simulink model "Udan_SOC"  (R2017b)
settings: Solver=FixedStepAuto  StartTime=0.0  StopTime=1000  FixedStep=0.1  RelTol=1e-3
values from neighbouring files (symbols this model uses):
  DenominatorOfIntegratorFactor = 100.0    [SOC_Stateflow.sldd]
  SOC_CalcSohLKT = 1.0    [SOC_Stateflow.sldd]
  SOC_CalcSOHTempLimit = 70.0    [SOC_Stateflow.sldd]
  SOC_CapPerCycle = 100.0    [SOC_Stateflow.sldd]
  SOC_CapTemp_HLimit = 200.0    [SOC_Stateflow.sldd]
  SOC_CapTemp_LLimit = 0.0    [SOC_Stateflow.sldd]
  Soc_ConfigInfo = 0    [SOC_Stateflow.sldd]
  SOC_DchgEndCalib = 0.0    [SOC_Stateflow.sldd]
  SOC_DiffVoltMin = 10.0    [SOC_Stateflow.sldd]
  SOC_DSOCJumpMax = 500.0    [SOC_Stateflow.sldd]
  SOC_EfficientHighLimit = 250.0    [SOC_Stateflow.sldd]
  SOC_EfficientLowLimit = 40.0    [SOC_Stateflow.sldd]
  SOC_EmptyAus = 0.0    [SOC_Stateflow.sldd]
  SOC_EnableOcv = 1.0    [SOC_Stateflow.sldd]
  SOC_END_CALIB_STATE : value not decoded    [SOC_Stateflow.sldd]
  SOC_HighRealSoc = 95.0    [SOC_Stateflow.sldd]
  SOC_LKTSohCycles = 0.0 1.0 10.0 20.0 30.0 40.0 50.0 60.0 70.0 80.0 90.0 100.0 110.0 120.0 130.0 140.0 150.0 160.0 170.0 180.0 190.0 200.0 210.0 220.0 230.0 240.0 250.0 260.0 270.0 280.0 290.0 300.0 310.0 320.0 330.0 340.0 350.0 360.0 370.0 380.0 390.0 400.0 410.0 420.0 430.0 440.0 450.0 460.0 470.0 480.0 490.0 500.0 510.0 520.0 530.0 540.0 550.0 560.0 570.0 580.0 590.0 600.0 610.0 620.0 630.0 640.0 650.0 660.0 670.0    [SOC_Stateflow.sldd]
  SOC_LKTSohTable = 1000.0 991.0 989.0 992.0 993.0 995.0 994.0 993.0 1000.0 997.0 1002.0 1000.0 992.0 1000.0 989.0 992.0 989.0 994.0 989.0 993.0 994.0 994.0 994.0 993.0 991.0 991.0 992.0 993.0 991.0 985.0 985.0 985.0 979.0 975.0 978.0 984.0 982.0 974.0 975.0 972.0 972.0 975.0 977.0 977.0 974.0 971.0 973.0 971.0 966.0 968.0 965.0 959.0 957.0 956.0 957.0 954.0 955.0 951.0 954.0 951.0 942.0 942.0 940.0 942.0 947.0 949.0    [SOC_Stateflow.sldd]
  SOC_LowRealSoc = 5.0    [SOC_Stateflow.sldd]
  SOC_NominalCap_AmS = 576000000.0    [SOC_Stateflow.sldd]
  SOC_NominalVol = 4000.0    [SOC_Stateflow.sldd]
  SOC_OCVTemp_HLimit = 106.0    [SOC_Stateflow.sldd]
  SOC_OCVTemp_LLimit = 29.0    [SOC_Stateflow.sldd]
  SOC_ShortCalibDSoc = 1.0    [SOC_Stateflow.sldd]
  SOC_SOCResolution = 10000.0    [SOC_Stateflow.sldd]
  SOC_SohCalcCapPercent = 8.0    [SOC_Stateflow.sldd]
  SOC_SohCalcHighLimit = 60.0    [SOC_Stateflow.sldd]
  SOC_SohCalcLowLimit = 10.0    [SOC_Stateflow.sldd]
  SOC_SohCalcMidLimit = 30.0    [SOC_Stateflow.sldd]
  SOC_SOHResolution = 1000.0    [SOC_Stateflow.sldd]
  SOC_State = <binary blob, 1163 chars, not shown>    [SOC_Stateflow.sldd]
  SOC_TempCap_CapBuffer : value not decoded    [SOC_Stateflow.sldd]
  SOC_TempCap_TempBuffer : value not decoded    [SOC_Stateflow.sldd]
  SocOcvCalib_ConfigInfo = 0.0    [SOC_Stateflow.sldd]
  SocOcvCalib_SocBuffer1 : value not decoded    [SOC_Stateflow.sldd]
  SocOcvCalib_TempBuffer : value not decoded    [SOC_Stateflow.sldd]
  SocOcvCalib_VoltageBuffer1 = 3300.0 3303.0 3305.0 3307.0 3310.0 3311.0 3313.0 3314.0 3316.0 3317.0 3319.0 3320.0 3322.0 3323.0 3325.0 3322.0 3323.0 3325.0 3310.0 3313.0 3315.0 3317.0 3320.0 3321.0 3323.0 3324.0 3326.0 3327.0 3329.0 3330.0 3332.0 3333.0 3335.0 3332.0 3333.0 3335.0 3320.0 3323.0 3325.0 3327.0 3330.0 3331.0 3333.0 3334.0 3336.0 3337.0 3339.0 3340.0 3342.0 3343.0 3345.0 3342.0 3343.0 3345.0 3330.0 3333.0 3335.0 3    [SOC_Stateflow.sldd]
  SOHCalibCycle = 10.0    [SOC_Stateflow.sldd]
undefined symbols (not defined in the file or in its folder): DatetimeM_GetReturnType, ParameterM_EeepParaIndexType, Soc_CumuLativeTypeType, SOC_EgthTempChgValue, Soc_EnergyBuffer, SOC_FithTempChgValue, SOC_FstSlowTempChgValue, SOC_FstTempChgValue, SOC_FthTempChgValue, SOC_MaxCap_AmS, SOC_SethTempChgValue, SOC_SixTempChgValue, SOC_SndSlowTempChgValue, SOC_SndTempChgValue, SOC_TrdSlowTempChgValue, SOC_TrdTempChgValue, SocDiagCalib_NoCalibReasonType
libraries: simulink x138, hdlsllib x24, dspindex x4
(part 9 of 10)

== matlab function Udan_SOC/SOC_Calculate/UdanSOCCalcn/LKTSOC/MATLAB Function2 ==
  data: cellTable input; enableOcv output; uCell input; diffVMin input; socBuffer input
function enableOcv = fcn(cellTable, uCell,diffVMin, socBuffer)
flag = uint8(0);
enableOcv = uint8(0);
for i = 1 : length(cellTable)-1
    if i == length(cellTable)
       flag = uint8(1);
    elseif uCell < cellTable(1)
           flag = uint8(1);
           break;
    else
           if cellTable(i)<=uCell && uCell < cellTable(i+1)
                break;
          end
    end
end
if flag < 1
    if i == 1 
        if cellTable(i+2) > cellTable(i+1) + uint16(diffVMin) && cellTable(i+1) > cellTable(i)+uint16(diffVMin) %% 压差大于10mv才认为区间有效
            flag = uint8(1);
        end
    elseif uCell >=cellTable(length(cellTable)) || socBuffer(i)>=10000
         flag = uint8(1);
    else
            if socBuffer(i+2)<=10000
                if cellTable(i+2) > cellTable(i+1) + uint16(diffVMin) && cellTable(i+1) > cellTable(i)+uint16(diffVMin) && cellTable(i) > cellTable(i-1)+uint16(diffVMin)
                    flag = uint8(1);
                end
            elseif socBuffer(i+1)<=10000
                if cellTable(i+1) > cellTable(i)+uint16(diffVMin) && cellTable(i) > cellTable(i-1)+uint16(diffVMin)
                    flag = uint8(1);
                end
            elseif socBuffer(i)<=10000
                if cellTable(i) > cellTable(i-1)+uint16(diffVMin)
                    flag = uint8(1);
                end
            else
                flag = uint8(1);
            end
    end
end

enableOcv = flag;

== matlab function Udan_SOC/SOC_Calculate/UdanSOCCalcn/Function-Call Subsystem4/Subsystem2/MATLAB Function2 ==
  data: input input; y output; bp input; table input
function y = interp_linear(input,bp,table)
data_type = class(table);
switch data_type
    case 'uint8'
        y = uint8(0);
    case 'uint16'
        y = uint16(0);
    case 'uint32'
        y = uint32(0);
end
if bp(1) == bp(2)
    y = table(2);
elseif length(bp) == length(table)
    if input <= bp(1)
        y = table(1);
    elseif input >= bp(end)
        y = table(end);
    else
        for i = 1 : length(bp)-1
            if input == bp(i)
                y = table(i);
                break;
            elseif input > bp(i) && input < bp(i+1)
                y = uint16(uint32(table(i)) - (uint32(table(i) - table(i+1)))*uint32((input-bp(i)))/uint32((bp(i+1)-bp(i))));
                break;
            else
            end
        end
    end
else
    msg = 'size dismatch';
    error(masg);
    y = 0;
end

== matlab function Udan_SOC/SOC_Calculate/UdanSOCCalcn/Function-Call Subsystem4/Subsystem2/MATLAB Function3 ==
  data: soh input; Cycles input; bp output; Table input; table output
function [bp,table] = fcn(soh, Cycles,Table)
    data_type = class(Table);
    uint8 index;
    index = GetSohLocationIndex(soh,Table);
    switch data_type
        case 'uint8'
            bp = uint8([Table(index+1) Table(index)]);
            table = GetDataType([Cycles(index) Cycles(index+1)]);
        case 'uint16'
            bp = uint16([Table(index+1) Table(index)]);
            table = GetDataType([Cycles(index) Cycles(index+1)]);
        case 'uint32'
            bp = uint32([Table(index+1) Table(index)]);
            table = GetDataType([Cycles(index) Cycles(index+1)]);
        otherwise
            bp = [ 0 0];
            table = [0 0];

    end
end
function ret = GetDataType(input)
    data_type1 = class(input);
    switch data_type1
        case 'uint8'
            ret = uint8([max(input) min(input)]);
        case 'uint16'
            ret = uint16([max(input) min(input)]);
        case 'uint32'
            ret = uint32([max(input) min(input)]);
        otherwise
            ret = [0 0];

    end
end

function index = GetSohLocationIndex(soh,sohTable)
    len = uint8(length(sohTable));
    i = uint8(0);
    index = uint8(1);
    if soh >= sohTable(1)
        index = uint8(1);
    elseif soh <= sohTable(len)
        index = len - 1;
    else
        for i = 1 : len - 1
            if soh <= sohTable(i) && soh>= sohTable(i+1)
                index = i;
                break;
            end
        end
    end
end

== stateflow chart Udan_SOC/SOC_Calculate/UdanSOCCalcn/CalcChgSOH/Subsystem/Chart2 ==
  state triggerflag=CalcDiff(subtrahend,minuend,diff) [function]
    (default) -> (junction 15)
    (junction 15) -> (junction 16) [order 1] : [subtrahend<=minuend]{delta=minuend-subtrahend;}
    (junction 16) -> (junction 17) [order 1] : [delta>diff]
    (junction 15) -> (junction 18) [order 2] : {delta=subtrahend-minuend;}
    (junction 16) -> (junction 22) [order 2] : {out=0;}
    (junction 17) -> (junction 23) : {out=-1;}
    (junction 18) -> (junction 19) [order 1] : [delta>diff]
    (junction 18) -> (junction 20) [order 2] : {out=0;}
    (junction 19) -> (junction 21) : {out=1;}
    (junction 21) -> (junction 20)
    (junction 22) -> (junction 21)
    (junction 23) -> (junction 22)
    (junction 20) -> (junction 24) : {triggerflag=out;}
  (default) -> (junction 52)
  (junction 52) -> (junction 53) [order 1] : [CalcDiff(CalcSOH,EEEPSOH,MaxDiff)==0&&...
      | CalcDiff(CalcSOH,EEEPSOH,MaxCal1)!=0]
  (junction 53) -> (junction 63) [order 1] : [CalcDiff(CalcSOH,EEEPSOH,MaxCal)==0&&...
      | CalcDiff(CalcSOH,EEEPSOH,MaxCal1)!=0]
  (junction 63) -> (junction 89) [order 1] : [CalcDiff(CalcSOH,EEEPSOH,MaxCal1)==1]
  (junction 52) -> (junction 58) [order 2] : {SohOut=EEEPSOH;}
  (junction 53) -> (junction 67) [order 2]
  (junction 63) -> (junction 65) [order 2] : {SohOut=EEEPSOH-5;
      | SOHWriteResult=1;}
  (junction 89) -> (junction 91) : {SohOut=EEEPSOH+5;
      | SOHWriteResult=1;}
  (junction 67) -> (junction 68) [order 1] : [CalcDiff(CalcSOH,EEEPSOH,MaxCal)==-1]
  (junction 67) -> (junction 61) [order 2] : {SohOut=EEEPSOH+10;
      | SOHWriteResult=1;}
  (junction 68) -> (junction 70) : {SohOut=EEEPSOH-10;
      | SOHWriteResult=1;}
  (junction 61) -> (junction 58)
  (junction 70) -> (junction 61)
  (junction 65) -> (junction 70)
  (junction 91) -> (junction 65)
  (junction 58) -> (junction 62)
  data: subtrahend function_input uint16; minuend function_input uint16; diff function_input int16; triggerflag function_output int8; delta local int16; out local int8; CalcSOH input; SOHWriteResult output uint8; SohOut output uint16; MaxDiff input; MaxCal input; MaxCal1 input; EEEPSOH input

== stateflow chart Udan_SOC/SOC_Calculate/UdanSOCCalcn/CalcDchgSOH/Subsystem/Chart1 ==
  state triggerflag=CalcDiff(subtrahend,minuend,diff) [function]
    (default) -> (junction 15)
    (junction 15) -> (junction 16) [order 1] : [subtrahend<=minuend]{delta=minuend-subtrahend;}
    (junction 16) -> (junction 17) [order 1] : [delta>diff]
    (junction 15) -> (junction 18) [order 2] : {delta=subtrahend-minuend;}
    (junction 16) -> (junction 22) [order 2] : {out=0;}
    (junction 17) -> (junction 23) : {out=-1;}
    (junction 18) -> (junction 19) [order 1] : [delta>diff]
    (junction 18) -> (junction 20) [order 2] : {out=0;}
    (junction 19) -> (junction 21) : {out=1;}
    (junction 21) -> (junction 20)
    (junction 22) -> (junction 21)
    (junction 23) -> (junction 22)
    (junction 20) -> (junction 24) : {triggerflag=out;}
  (default) -> (junction 52)
  (junction 52) -> (junction 53) [order 1] : [CalcDiff(CalcSOH,EEEPSOH,MaxDiff)==0&&...
      | CalcDiff(CalcSOH,EEEPSOH,MaxCal1)!=0]
  (junction 53) -> (junction 63) [order 1] : [CalcDiff(CalcSOH,EEEPSOH,MaxCal)==0&&...
      | CalcDiff(CalcSOH,EEEPSOH,MaxCal1)!=0]
  (junction 63) -> (junction 89) [order 1] : [CalcDiff(CalcSOH,EEEPSOH,MaxCal1)==1]
  (junction 52) -> (junction 58) [order 2] : {SohOut=EEEPSOH;}
  (junction 53) -> (junction 67) [order 2]
  (junction 63) -> (junction 65) [order 2] : {SohOut=EEEPSOH-5;
      | SOHWriteResult=1;}
  (junction 89) -> (junction 91) : {SohOut=EEEPSOH+5;
      | SOHWriteResult=1;}
  (junction 67) -> (junction 68) [order 1] : [CalcDiff(CalcSOH,EEEPSOH,MaxCal)==-1]
  (junction 67) -> (junction 61) [order 2] : {SohOut=EEEPSOH+10;
      | SOHWriteResult=1;}
  (junction 68) -> (junction 70) : {SohOut=EEEPSOH-10;
      | SOHWriteResult=1;}
  (junction 61) -> (junction 58)
  (junction 70) -> (junction 61)
  (junction 65) -> (junction 70)
  (junction 91) -> (junction 65)
  (junction 58) -> (junction 62)
  data: subtrahend function_input uint16; minuend function_input uint16; diff function_input int16; triggerflag function_output int8; delta local int16; out local int8; CalcSOH input; SOHWriteResult output uint8; SohOut output uint16; MaxDiff input; MaxCal input; MaxCal1 input; EEEPSOH input

== stateflow chart Udan_SOC/SOC_Calculate/UdanSOCCalcn/CalclnCore ==
  state InitState
    en:
    SOC_State=SOC_STATE_INIT;
    InitSOC;
    du:
    Timer.T2.Run(250);
    InitSOC;
    ex:
    Timer.T2.Clear();
  state Timer [function]
    state T2 [function]
      state Run(Cycle) [function]
        (default) -> (junction 285)
        (junction 285) -> (junction 286) [order 1] : [tick==0]{Timetick=Cycle/10;tick=1}
        (junction 286) -> (junction 287)
        (junction 285) -> (junction 287) [order 2]
        (junction 287) -> (junction 288) [order 2] : {Timetick = Timetick - 1}
        (junction 287) -> (junction 289) [order 1] : [Timetick==0]{TimerOut=1}
      state Clear [function]
        (default) -> (junction 297)
        (junction 297) -> (junction 298) : {tick=0;TimerOut= uint16(0);}
  state y=ABS(u) [function]
    (default) -> (junction 364)
    (junction 364) -> (junction 366) [order 1] : [u<=0]
    (junction 366) -> (junction 367) : {Local=-u;}
    (junction 364) -> (junction 367) [order 2] : {Local=u}
    (junction 367) -> (junction 368) : {y=Local;}
  state CalcDchSOH1
    en:
    SohCond=1;
    SOC_State=SOC_STATE_OCV_LONG;
    LookUpOcvTable;
    WriteOCVTime;
  state OcvSoc
    en:
    SOC_State=SOC_STATE_OCV;
    SohCond=1;
    LookUpOcvTable;
    WriteOCVTime;
  state EmptyCalib
    en:
    SOC_State=SOC_STATE_EMPTY;
    CalibEmptySOC;
    EmptyCalibFlag=1;
  state CalcSOC
    en:
    SOC_State=SOC_STATE_INTEGRATE;
    SOCIntegrate;
    DeltaOcvTime=int32(NowTime-LastTime);
    du:
    DeltaOcvTime=int32(NowTime-LastTime);
    SOCIntegrate;
    CalcSOC -> CalcSOC [order 1] : [(NowTime<LastTime)||...
        | (largeCurrentFlag==1&&DeltaOcvTime>checkCycle&&...
        | OSTime>powerOnDelay)]
        | {WriteOCVTime;
        | OCVTimeChangeFlag=1;}
    CalcSOC -> CalcSOC [order 2] : [(NowTime-OcvCalibTime)>30&&...
        | (ABS(Current)>=CurrentMax)&&...
        | (SohCond==1)&&(Current<0)&&largeCurrentFlag==0]
        | {OcvCalibTime=NowTime;SohCond=0;}
  state CalcDchSOH
    en:
    SOC_State=SOC_STATE_DCHGSOH;
    SohCond=1;
    LookUpOcvTable;
    CalcDchgSOH;
    WriteOCVTime;
  state CalcnChgSOH
    en:
    SOC_State=SOC_STATE_SOH;
    SohCond=0;
    CalcChgSOH;
  state MannualCalib
    en:
    SOC_State=SOC_STATE_INIT;
    InitSOC;
  state FullCalib
    en:
    SOC_State=SOC_STATE_FULL;
    CalibFullSOC;
    FullCalibFlag=1;
  (default) -> InitState
  InitState -> CalcDchSOH1 [order 1] : [OSTime>powerOnDelay&&ABS(Current)<=CurrentMax&&...
      | RtcTimeIsOk&&BmuStateIsOk&&LongBatOffTimeOk==1]
  InitState -> OcvSoc [order 2] : [(BatOffTimeOk==1)&&BmuStateIsOk==1&&...
      | ABS(Current)<=CurrentMax&&RtcTimeIsOk&&...
      | OSTime>powerOnDelay]
  InitState -> CalcSOC [order 3]
  CalcSOC -> CalcDchSOH1 [order 1] : [OSTime>powerOnDelay&&ABS(Current)<=CurrentMax&&...
      | RtcTimeIsOk&&BmuStateIsOk&&LongBatOffTimeOk==1&&...
      | largeCurrentFlag==0&&EnableOcv]
  CalcDchSOH1 -> CalcSOC
  CalcSOC -> OcvSoc [order 2] : [(BatOffTimeOk==1)&&BmuStateIsOk==1&&...
      | ABS(Current)<=CurrentMax&&RtcTimeIsOk&&...
      | OSTime>powerOnDelay&&largeCurrentFlag==0&&...
      | EnableOcv]
  OcvSoc -> CalcSOC
  CalcSOC -> CalcDchSOH [order 4] : [(SohTimeDiffOk==1||...
      | BatOffTimeOk==1||LongBatOffTimeOk)&&...
      | SohCond==0&&BmuStateIsOk==1&&...
      | ABS(Current)<=CurrentMax&&RtcTimeIsOk&&...
      | OSTime>powerOnDelay&&largeCurrentFlag==0&&...
      | EnableOcv]
  EmptyCalib -> CalcSOC : [EmptyDchgFlag==0]
  CalcDchSOH -> CalcSOC
  CalcSOC -> EmptyCalib [order 5] : [EmptyDchgFlag==1]
  MannualCalib -> CalcSOC
  CalcSOC -> MannualCalib [order 6] : [SocCalibFlag==1]
  CalcSOC -> FullCalib [order 3] : [FullChgFns==1]
  FullCalib -> CalcSOC [order 2] : [FullChgFns==0]
  CalcnChgSOH -> CalcSOC
  FullCalib -> CalcnChgSOH [order 1] : [SohCond==1&&...
      | EnableOcv]
  data: Cycle function_input uint16; tick local uint8; Timetick local uint8; u function_input int16; y function_output int16; Local local int16; RtcTimeIsOk input; NowTime input; BmuStateIsOk input; LongBatOffTimeOk input; BatOffTimeOk input; SohTimeDiffOk input; SohCond local boolean; CurrentMax input; checkCycle input; CalibCycle input; Current input; DeltaOcvTime local int32; LastTime input; FullChgFns input; SOC_State output Enum: SOC_State; TimerOut local boolean; EmptyDchgFlag input; SocCalibFlag input; EmptyCalibFlag local boolean; IsCharging input; OCVTimeChangeFlag local boolean; OcvCalibTime local uint32; FullCalibFlag local uint8; powerOnDelay input; OSTime input; largeCurrentFlag input; EnableOcv input
  events: InitSOC output FUNCTION_CALL_EVENT; LookUpOcvTable output FUNCTION_CALL_EVENT; SOCIntegrate output FUNCTION_CALL_EVENT; CalibFullSOC output FUNCTION_CALL_EVENT; CalibEmptySOC output FUNCTION_CALL_EVENT; CalcDchgSOH output FUNCTION_CALL_EVENT; WriteOCVTime output FUNCTION_CALL_EVENT; CalcChgSOH output FUNCTION_CALL_EVENT

== stateflow chart Udan_SOC/SOC_Calculate/UdanSOCCalcn/CalcnLeftChargeTime/CalcLeftTime/CalcLeftTime ==
  state ret=CalcEvyTime(TargetCap,NowCap,Current) [function]
    (default) -> (junction 27)
    (junction 27) -> (junction 33) [order 3] : {ret=(TargetCap-NowCap)/((uint32(Current)*100));}
    (junction 27) -> (junction 33) [order 1] : [Current==0]{ret=18*3600;}
    (junction 27) -> (junction 33) [order 2] : [Current == 65535]{ret = 0;}%无效电流
  state y=abs(in1,in2) [function]
    (default) -> (junction 83)
    (junction 83) -> (junction 88) [order 1] : [in1<in2]
    (junction 88) -> (junction 89) : {y=in2-in1;}
    (junction 83) -> (junction 89) [order 2] : {y=in1-in2;}
    (junction 89) -> (junction 90)
  state ret = diagPercentIsValid(Percent1,Percent2) [function]
    (default) -> (junction 115)
    (junction 115) -> (junction 120) [order 1] : [Percent2~=65535]{ret=Percent2;}
    (junction 115) -> (junction 120) [order 2] : {ret=Percent1;}
  (default) -> (junction 15) : {result=0;}
  (junction 15) -> (junction 16) [order 1] : [DleftCap>=NominalCap]
  (junction 16) -> (junction 24) : {TimeOut=0;}
  (junction 15) -> (junction 17) [order 2]
  (junction 64) -> (junction 18) [order 2] : {LocalCur=PackCur;}
  (junction 64) -> (junction 18) [order 1] : [PackCur<80]
      | {LocalCur=Cur1;}
  (junction 17) -> (junction 64) [order 1] : [DleftCap<FstDecPnt]
  (junction 18) -> (junction 79) : {ValidSndDecPnt = diagPercentIsValid(FstDecPnt,SndDecPnt);
      | ValidTrdDecPnt = diagPercentIsValid(ValidSndDecPnt,TrdDecPnt);
      | ValidCur2=diagPercentIsValid(uint32(Cur1),uint32(Cur2));
      | ValidCur3=diagPercentIsValid(uint32(ValidCur2),uint32(Cur3));
      | ValidCur4=diagPercentIsValid(uint32(ValidCur3),uint32(Cur4));
      | TimeOut=CalcEvyTime(FstDecPnt,DleftCap,uint16(LocalCur))+...
      |                  CalcEvyTime(ValidSndDecPnt,FstDecPnt,uint16(ValidCur2))+...
      |                  CalcEvyTime(ValidTrdDecPnt,ValidSndDecPnt,uint16(ValidCur3))+...
      |                  CalcEvyTime(NominalCap,ValidTrdDecPnt,uint16(ValidCur4));}
  (junction 17) -> (junction 19) [order 2]
  (junction 67) -> (junction 20) [order 2] : {LocalCur=PackCur;}
  (junction 19) -> (junction 67) [order 1] : [DleftCap<SndDecPnt &&...
      | SndDecPnt ~= 65535]
  (junction 67) -> (junction 20) [order 1] : [PackCur<80]
      | {LocalCur=Cur2;}
  (junction 19) -> (junction 35) [order 2]
  (junction 20) -> (junction 95) : {TimeOut=CalcEvyTime(SndDecPnt,DleftCap,LocalCur)+...
      | CalcEvyTime(TrdDecPnt,SndDecPnt,Cur3)+...
      | CalcEvyTime(NominalCap,TrdDecPnt,Cur4)}
  (junction 70) -> (junction 36) [order 2] : {LocalCur=PackCur;}
  (junction 35) -> (junction 70) [order 1] : [DleftCap<TrdDecPnt &&...
      | SndDecPnt ~= 65535]
  (junction 70) -> (junction 36) [order 1] : [PackCur<80]
      | {LocalCur=Cur3;}
  (junction 35) -> (junction 73) [order 3] : {LocalCur=PackCur;}
  (junction 36) -> (junction 98) : {TimeOut=CalcEvyTime(TrdDecPnt,DleftCap,LocalCur)+...
      | CalcEvyTime(NominalCap,TrdDecPnt,Cur4)}
  (junction 35) -> (junction 73) [order 2] : [PackCur<80]
      | {
      | ValidCur2=diagPercentIsValid(uint32(Cur1),uint32(Cur2));
      | ValidCur3=diagPercentIsValid(uint32(ValidCur2),uint32(Cur3));
      | ValidCur4=diagPercentIsValid(uint32(ValidCur3),uint32(Cur4));
      | LocalCur=ValidCur4;
      | }
  (junction 79) -> (junction 23) [order 2]
  (junction 79) -> (junction 23) [order 1] : [abs(Cur1,PackCur)<=50]{result=1;}
  (junction 95) -> (junction 22) [order 2]
  (junction 95) -> (junction 22) [order 1] : [abs(Cur1,PackCur)<=50]{result=1;}
  (junction 98) -> (junction 38) [order 2]
  (junction 73) -> (junction 101) : {TimeOut=CalcEvyTime(NominalCap,DleftCap,LocalCur)}
  (junction 98) -> (junction 38) [order 1] : [abs(Cur1,PackCur)<=50]{result=1;}
  (junction 101) -> (junction 21) [order 2]
  (junction 101) -> (junction 21) [order 1] : [abs(Cur1,PackCur)<=50]{result=1;}
  (junction 38) -> (junction 21)
  (junction 22) -> (junction 38)
  (junction 23) -> (junction 22)
  (junction 24) -> (junction 23)
  (junction 21) -> (junction 25) [order 2]
  (junction 21) -> (junction 25) [order 1] : [TimeOut>18*3600]{TimeOut=18*3600;}
  (junction 25) -> (junction 76)
  data: TargetCap function_input uint32; NowCap function_input uint32; Current function_input uint16; ret function_output uint32; in1 function_input uint16; in2 function_input int16; y function_output int16; ret function_output uint32; Percent1 function_input uint32; Percent2 function_input uint32; DleftCap input; PackCur input; NominalCap input; FstDecPnt input; SndDecPnt input; TrdDecPnt input; Cur1 input; Cur2 input; Cur3 input; Cur4 input; TimeOut output uint32; LocalCur local int16; result output boolean; ValidSndDecPnt local uint32; ValidTrdDecPnt local uint32; ValidCur2 local uint16; ValidCur3 local uint16; ValidCur4 local uint16

== stateflow chart Udan_SOC/SOC_Calculate/UdanSOCCalcn/CalcnLeftChargeTime/CalcLeftTime/SelectChgCurrent ==
  (default) -> (junction 11)
  (junction 11) -> (junction 12) [order 1] : [BatTemp<=40]
  (junction 11) -> (junction 13) [order 2]
  (junction 12) -> (junction 17) : {ChgCurOut=FstChgCur;}
  (junction 13) -> (junction 14) [order 2] : [BatTemp<=50]
  (junction 13) -> (junction 19) [order 1]
  (junction 14) -> (junction 16) : {ChgCurOut=SndChgCur;}
  (junction 19) -> (junction 20) [order 1] : [BatTemp<=60]
  (junction 19) -> (junction 24) [order 2]
  (junction 20) -> (junction 22) : {ChgCurOut=TrdChgCur;}
  (junction 24) -> (junction 26) [order 1] : [BatTemp<=75]
  (junction 24) -> (junction 31) [order 2]
  (junction 26) -> (junction 28) : {ChgCurOut=FthChgCur;}
  (junction 31) -> (junction 33) [order 1] : [BatTemp<=95]
  (junction 31) -> (junction 38) [order 2]
  (junction 33) -> (junction 34) : {ChgCurOut=FithChgCur;}
  (junction 38) -> (junction 40) [order 1] : [BatTemp<=100]
  (junction 38) -> (junction 45) [order 2]
  (junction 40) -> (junction 42) : {ChgCurOut=SixChgCur;}
  (junction 45) -> (junction 47) [order 1] : [BatTemp<=110]
  (junction 45) -> (junction 15) [order 2] : {ChgCurOut=EgthTempChgValue;}
  (junction 47) -> (junction 49) : {ChgCurOut=SevenChgCur;}
  (junction 49) -> (junction 15)
  (junction 42) -> (junction 49)
  (junction 34) -> (junction 42)
  (junction 28) -> (junction 34)
  (junction 22) -> (junction 28)
  (junction 16) -> (junction 22)
  (junction 17) -> (junction 16)
  (junction 15) -> (junction 18)
  data: BatTemp input; FstChgCur input; SndChgCur input; TrdChgCur input; FthChgCur input; FithChgCur input; SixChgCur input; SevenChgCur input; EgthTempChgValue input; ChgCurOut output Bus: SOC_ChgCurrentType

== stateflow chart Udan_SOC/SOC_Calculate/UdanSOCCalcn/CalcnLeftChargeTime/CalcLeftTime/SelectChgCurrent1 ==
  (default) -> (junction 11)
  (junction 11) -> (junction 12) [order 1] : [BatTemp<=40]
  (junction 11) -> (junction 13) [order 2]
  (junction 12) -> (junction 17) : {ChgCurOut=FstChgCur;}
  (junction 13) -> (junction 14) [order 2] : [BatTemp<=50]
  (junction 13) -> (junction 19) [order 1]
  (junction 14) -> (junction 16) : {ChgCurOut=SndChgCur;}
  (junction 19) -> (junction 20) [order 1] : [BatTemp<=60]
  (junction 19) -> (junction 24) [order 2]
  (junction 20) -> (junction 22) : {ChgCurOut=TrdChgCur;}
  (junction 24) -> (junction 26) [order 1] : [BatTemp<=75]
  (junction 24) -> (junction 31) [order 2]
  (junction 26) -> (junction 28) : {ChgCurOut=FthChgCur;}
  (junction 31) -> (junction 33) [order 1] : [BatTemp<=95]
  (junction 31) -> (junction 38) [order 2]
  (junction 33) -> (junction 34) : {ChgCurOut=FithChgCur;}
  (junction 38) -> (junction 40) [order 1] : [BatTemp<=100]
  (junction 38) -> (junction 45) [order 2]
  (junction 40) -> (junction 42) : {ChgCurOut=SixChgCur;}
  (junction 45) -> (junction 47) [order 1] : [BatTemp<=110]
  (junction 45) -> (junction 15) [order 2] : {ChgCurOut=EgthTempChgValue;}
  (junction 47) -> (junction 49) : {ChgCurOut=SevenChgCur;}
  (junction 49) -> (junction 15)
  (junction 42) -> (junction 49)
  (junction 34) -> (junction 42)
  (junction 28) -> (junction 34)
  (junction 22) -> (junction 28)
  (junction 16) -> (junction 22)
  (junction 17) -> (junction 16)
  (junction 15) -> (junction 18)
  data: BatTemp input; FstChgCur input; SndChgCur input; TrdChgCur input; FthChgCur input; FithChgCur input; SixChgCur input; SevenChgCur input; EgthTempChgValue input; ChgCurOut output Bus: SOC_ChgCurrentType

== stateflow chart Udan_SOC/SOC_Calculate/UdanSOCCalcn/CalcnLeftChargeTime/CalcLeftTime1/CalcLeftTime ==
  state ret=CalcEvyTime(TargetCap,NowCap,Current) [function]
    (default) -> (junction 27)
    (junction 27) -> (junction 33) [order 3] : {ret=(TargetCap-NowCap)/((uint32(Current)*100));}
    (junction 27) -> (junction 33) [order 1] : [Current==0]{ret=18*3600;}
    (junction 27) -> (junction 33) [order 2] : [Current == 65535]{ret = 0;}%无效电流
  state y=abs(in1,in2) [function]
    (default) -> (junction 83)
    (junction 83) -> (junction 88) [order 1] : [in1<in2]
    (junction 88) -> (junction 89) : {y=in2-in1;}
    (junction 83) -> (junction 89) [order 2] : {y=in1-in2;}
    (junction 89) -> (junction 90)
  state ret = diagPercentIsValid(Percent1,Percent2) [function]
    (default) -> (junction 115)
    (junction 115) -> (junction 120) [order 1] : [Percent2~=65535]{ret=Percent2;}
    (junction 115) -> (junction 120) [order 2] : {ret=Percent1;}
  (default) -> (junction 15) : {result=0;}
  (junction 15) -> (junction 16) [order 1] : [DleftCap>=NominalCap]
  (junction 16) -> (junction 24) : {TimeOut=0;}
  (junction 15) -> (junction 17) [order 2]
  (junction 64) -> (junction 18) [order 2] : {LocalCur=PackCur;}
  (junction 64) -> (junction 18) [order 1] : [PackCur<30]
      | {LocalCur=Cur1;}
  (junction 17) -> (junction 64) [order 1] : [DleftCap<FstDecPnt]
  (junction 18) -> (junction 79) : {ValidSndDecPnt = diagPercentIsValid(FstDecPnt,SndDecPnt);
      | ValidTrdDecPnt = diagPercentIsValid(ValidSndDecPnt,TrdDecPnt);
      | ValidCur2=diagPercentIsValid(uint32(Cur1),uint32(Cur2));
      | ValidCur3=diagPercentIsValid(uint32(ValidCur2),uint32(Cur3));
      | ValidCur4=diagPercentIsValid(uint32(ValidCur3),uint32(Cur4));
      | TimeOut=CalcEvyTime(FstDecPnt,DleftCap,uint16(LocalCur))+...
      |                  CalcEvyTime(ValidSndDecPnt,FstDecPnt,uint16(ValidCur2))+...
      |                  CalcEvyTime(ValidTrdDecPnt,ValidSndDecPnt,uint16(ValidCur3))+...
      |                  CalcEvyTime(NominalCap,ValidTrdDecPnt,uint16(ValidCur4));}
  (junction 17) -> (junction 19) [order 2]
  (junction 67) -> (junction 20) [order 2] : {LocalCur=PackCur;}
  (junction 19) -> (junction 67) [order 1] : [DleftCap<SndDecPnt &&...
      | SndDecPnt ~= 65535]
  (junction 67) -> (junction 20) [order 1] : [PackCur<30]
      | {LocalCur=Cur2;}
  (junction 19) -> (junction 35) [order 2]
  (junction 20) -> (junction 95) : {TimeOut=CalcEvyTime(SndDecPnt,DleftCap,LocalCur)+...
      | CalcEvyTime(TrdDecPnt,SndDecPnt,Cur3)+...
      | CalcEvyTime(NominalCap,TrdDecPnt,Cur4)}
  (junction 70) -> (junction 36) [order 2] : {LocalCur=PackCur;}
  (junction 35) -> (junction 70) [order 1] : [DleftCap<TrdDecPnt &&...
      | SndDecPnt ~= 65535]
  (junction 70) -> (junction 36) [order 1] : [PackCur<30]
      | {LocalCur=Cur3;}
  (junction 35) -> (junction 73) [order 3] : {LocalCur=PackCur;}
  (junction 36) -> (junction 98) : {TimeOut=CalcEvyTime(TrdDecPnt,DleftCap,LocalCur)+...
      | CalcEvyTime(NominalCap,TrdDecPnt,Cur4)}
  (junction 35) -> (junction 73) [order 2] : [PackCur<30]
      | {
      | ValidCur2=diagPercentIsValid(uint32(Cur1),uint32(Cur2));
      | ValidCur3=diagPercentIsValid(uint32(ValidCur2),uint32(Cur3));
      | ValidCur4=diagPercentIsValid(uint32(ValidCur3),uint32(Cur4));
      | LocalCur=ValidCur4;
      | }
  (junction 79) -> (junction 23) [order 2]
  (junction 79) -> (junction 23) [order 1] : [abs(Cur1,PackCur)<=50]{result=1;}
  (junction 95) -> (junction 22) [order 2]
  (junction 95) -> (junction 22) [order 1] : [abs(Cur1,PackCur)<=50]{result=1;}
  (junction 98) -> (junction 38) [order 2]
  (junction 73) -> (junction 101) : {TimeOut=CalcEvyTime(NominalCap,DleftCap,LocalCur)}
  (junction 98) -> (junction 38) [order 1] : [abs(Cur1,PackCur)<=50]{result=1;}
  (junction 101) -> (junction 21) [order 2]
  (junction 101) -> (junction 21) [order 1] : [abs(Cur1,PackCur)<=50]{result=1;}
  (junction 38) -> (junction 21)
  (junction 22) -> (junction 38)
  (junction 23) -> (junction 22)
  (junction 24) -> (junction 23)
  (junction 21) -> (junction 25) [order 2]
  (junction 21) -> (junction 25) [order 1] : [TimeOut>18*3600]{TimeOut=18*3600;}
  (junction 25) -> (junction 76)
  data: TargetCap function_input uint32; NowCap function_input uint32; Current function_input uint16; ret function_output uint32; in1 function_input uint16; in2 function_input int16; y function_output int16; ret function_output uint32; Percent1 function_input uint32; Percent2 function_input uint32; DleftCap input; PackCur input; NominalCap input; FstDecPnt input; SndDecPnt input; TrdDecPnt input; Cur1 input; Cur2 input; Cur3 input; Cur4 input; TimeOut output uint32; LocalCur local int16; result output boolean; ValidSndDecPnt local uint32; ValidTrdDecPnt local uint32; ValidCur2 local uint16; ValidCur3 local uint16; ValidCur4 local uint16

== stateflow chart Udan_SOC/SOC_Calculate/UdanSOCCalcn/CalcnLeftChargeTime/CalcLeftTime1/SelectChgCurrent ==
  (default) -> (junction 11)
  (junction 11) -> (junction 12) [order 1] : [BatTemp<40]
  (junction 11) -> (junction 13) [order 2]
  (junction 12) -> (junction 17) : {ChgCurOut=FstChgCur;}
  (junction 13) -> (junction 14) [order 1] : [BatTemp<100]
  (junction 13) -> (junction 15) [order 2] : {ChgCurOut=TrdChgCur;}
  (junction 14) -> (junction 16) : {ChgCurOut=SndChgCur;}
  (junction 16) -> (junction 15)
  (junction 17) -> (junction 16)
  (junction 15) -> (junction 18)
  data: BatTemp input; FstChgCur input; SndChgCur input; TrdChgCur input; ChgCurOut output Bus: SOC_ChgCurrentType

== stateflow chart Udan_SOC/SOC_Calculate/UdanSOCCalcn/CalcnLeftChargeTime/CalcLeftTime1/SelectChgCurrent1 ==
  (default) -> (junction 11)
  (junction 11) -> (junction 12) [order 1] : [BatTemp<40]
  (junction 11) -> (junction 13) [order 2]
  (junction 12) -> (junction 17) : {ChgCurOut=FstChgCur;}
  (junction 13) -> (junction 14) [order 1] : [BatTemp<100]
  (junction 13) -> (junction 15) [order 2] : {ChgCurOut=TrdChgCur;}
  (junction 14) -> (junction 16) : {ChgCurOut=SndChgCur;}
  (junction 16) -> (junction 15)
  (junction 17) -> (junction 16)
  (junction 15) -> (junction 18)
  data: BatTemp input; FstChgCur input; SndChgCur input; TrdChgCur input; ChgCurOut output Bus: SOC_ChgCurrentType

== stateflow chart Udan_SOC/SOC_Calculate/UdanSOCCalcn/CalcnLeftChargeTime/DiagDrop1/DiagDropCore ==
  state triggerflag=CalcDiff(subtrahend,minuend,diff) [function]
    (default) -> (junction 27)
    (junction 27) -> (junction 30) [order 1] : [subtrahend<=minuend]{delta=minuend-subtrahend;}
    (junction 30) -> (junction 45) [order 1] : [delta>diff]
    (junction 27) -> (junction 46) [order 2] : {delta=subtrahend-minuend;}
    (junction 30) -> (junction 51) [order 2] : {out=0;}
    (junction 45) -> (junction 49) : {out=-1;}
    (junction 46) -> (junction 47) [order 1] : [delta>diff]
    (junction 46) -> (junction 32) [order 2] : {out=0;}
    (junction 47) -> (junction 54) : {out=1;}
    (junction 54) -> (junction 32)
    (junction 51) -> (junction 54)
    (junction 49) -> (junction 51)
    (junction 32) -> (junction 44) : {triggerflag=out;}
  state IncTimer
    en:
    CurState=1;
    IncTimer -> IncTimer [order 1] : [NowTime-LocalTime>=OutUpdateTick]
        | {CurrentSend=LastCurrentSend+increaseStep;
        | LocalTime=NowTime;}
  state InitState
    en:
    CurrentSend=CurrentOut;
    CurState=0;
  state DecTimer
    en:
    CurState=2;
    DecTimer -> DecTimer [order 1] : [NowTime-LocalTime>=OutUpdateTick]
        | {CurrentSend=LastCurrentSend-decreaseStep;LocalTime=NowTime;}
  (default) -> (junction 15) [commented out] : {result=LastState;}
  (junction 16) -> (junction 68) [commented out] : [CalcDiff(CurrentOut,LastCurrentSend,decreaseStep)==-1||...
      | CalcDiff(CurrentOut,LastCurrentSend,increaseStep)==1]
  (junction 68) -> (junction 124) [commented out] : [CalcDiff(CurrentOut,LastCurrentSend,increaseStep)==1]
  (junction 15) -> (junction 16) [commented out] : [result==0]
  (junction 16) -> (junction 24) [commented out] : {Current=CurrentOut;}
  (junction 68) -> (junction 69) [commented out] : {
      |  result=1;
      |  CurTime=uint16(NowTime&65535);
      | Current=LastCurrentSend;}
  (junction 124) -> (junction 126) [commented out] : {
      |  result=2;
      |  CurTime=uint16(NowTime&65535);
      | Current=LastCurrentSend;}
  (junction 15) -> (junction 133) [commented out]
  (junction 106) -> (junction 108) [commented out] : [CalcDiff(CurrentOut,LastCurrentSend,decreaseStep)~=-1]
  (junction 133) -> (junction 106) [commented out] : [LastState==1]
  (junction 106) -> (junction 113) [commented out] : [LastTime>=uint16(NowTime&65535)]
      | {diffTime=uint16(NowTime&65535)+65535-LastTime;}
  (junction 108) -> (junction 110) [commented out] : {result=0;
      | Current=LastCurrentSend}
  (junction 133) -> (junction 142) [commented out]
  (junction 106) -> (junction 113) [commented out] : {diffTime=uint16(NowTime&65535)-LastTime;}
  (junction 142) -> (junction 144) [commented out] : [CalcDiff(CurrentOut,LastCurrentSend,increaseStep)~=1]
  (junction 113) -> (junction 118) [commented out] : [diffTime>=OutUpdateTick]
  (junction 142) -> (junction 150) [commented out] : [LastTime>=uint16(NowTime&65535)]
      | {diffTime=uint16(NowTime&65535)+65535-LastTime;}
  (junction 142) -> (junction 150) [commented out] : {diffTime=uint16(NowTime&65535)-LastTime;}
  (junction 144) -> (junction 146) [commented out] : {result=0;
      | Current=LastCurrentSend}
  (junction 113) -> (junction 136) [commented out] : {Current=LastCurrentSend;}
  (junction 118) -> (junction 120) [commented out] : {result=0;
      | Current=LastCurrentSend-decreaseStep;}
  (junction 150) -> (junction 151) [commented out] : [diffTime>=OutUpdateTick]
  (default) -> (junction 210)
  (junction 150) -> (junction 139) [commented out] : {Current=LastCurrentSend;}
  (junction 151) -> (junction 152) [commented out] : {result=0;
      | Current=LastCurrentSend+increaseStep;}
  (junction 210) -> (junction 212) [order 1] : [CalcDiff(CurrentOut,LastCurrentSend,decreaseStep)==-1||...
      | CalcDiff(CurrentOut,LastCurrentSend,increaseStep)==1]
  InitState -> (junction 210) : [CalcDiff(CurrentOut,LastCurrentSend,decreaseStep)==-1||...
      | CalcDiff(CurrentOut,LastCurrentSend,increaseStep)==1]
  (junction 210) -> InitState [order 2]
  (junction 152) -> (junction 139) [commented out]
  (junction 146) -> (junction 152) [commented out]
  (junction 136) -> (junction 146) [commented out]
  (junction 132) -> (junction 136) [commented out]
  (junction 120) -> (junction 132) [commented out]
  (junction 69) -> (junction 24) [commented out]
  (junction 126) -> (junction 69) [commented out]
  (junction 110) -> (junction 120) [commented out]
  (junction 24) -> (junction 110) [commented out]
  (junction 139) -> (junction 25) [commented out] : {CurrentSend=Current;
      | CurState=result;}
  (junction 212) -> IncTimer [order 1] : [CalcDiff(CurrentOut,LastCurrentSend,increaseStep)==1]
      | {LocalTime=NowTime;  CurrentSend=LastCurrentSend+increaseStep;}
  (junction 212) -> DecTimer [order 2] : {LocalTime=NowTime;
      |  CurrentSend=LastCurrentSend-decreaseStep;}
  IncTimer -> DecTimer [order 2] : [CalcDiff(CurrentOut,LastCurrentSend,decreaseStep)==-1]
      | {LocalTime=NowTime;
      |  CurrentSend=LastCurrentSend-decreaseStep;}
  IncTimer -> InitState [order 1] : [CalcDiff(CurrentOut,LastCurrentSend,increaseStep)==0]
  DecTimer -> IncTimer [order 2] : [CalcDiff(CurrentOut,LastCurrentSend,increaseStep)==1]{CurrentSend=LastCurrentSend+increaseStep;
      | LocalTime=NowTime;}
  DecTimer -> InitState [order 1] : [CalcDiff(CurrentOut,LastCurrentSend,decreaseStep)==0]
  data: subtrahend function_input uint16; minuend function_input uint16; diff function_input uint16; triggerflag function_output int8; delta local int16; out local int8; CurrentOut input; NowTime input; decreaseStep input; increaseStep input; OutUpdateTick input; LastCurrentSend input uint32; CurrentSend output uint32; MaxVariantPower local uint32; result local uint8; Current local uint32; CurState output uint8; LastState input uint8; CurTime output uint16; LastTime input uint16; diffTime local uint32; LocalTime local uint32; LocalCurrentSend local uint32

== stateflow chart Udan_SOC/SOC_Calculate/UdanSOCCalcn/CapAdder1/Chart ==
  state ChgCalibInit
    en:
    SelectedIndex=0;
  state Timer [function]
    state T2 [function]
      state Run(Cycle,Cond) [function]
        (default) -> (junction 9)
        (junction 9) -> (junction 10) [order 2] : [tick==0]{Timetick=Cycle/250-1;tick=1}
        (junction 10) -> (junction 11)
        (junction 9) -> (junction 13) [order 1] : [Cond==0]{tick=0;TimerOut=0;}
        (junction 9) -> (junction 11) [order 3]
        (junction 11) -> (junction 12) [order 2] : {Timetick = Timetick - 1}
        (junction 11) -> (junction 13) [order 1] : [Timetick==0]{TimerOut=1}
        (junction 13) -> (junction 56)
      state Clear [function]
        (default) -> (junction 21)
        (junction 21) -> (junction 22) : {tick=0;TimerOut= uint16(0);}
  state ChgCalibDelay
    en:
    SelectedIndex=0;
    du:
    Timer.T2.Run(5000,LKTDecide());
    ex:
    Timer.T2.Clear();
  state LKTFlag=LKTDecide [function]
    (default) -> (junction 44)
    (junction 44) -> (junction 45) [order 1] : [BatTemp>=Table1TempLow&&...
        | BatTemp<Table1TempHigh&&...
        | BatUCell>=Table1UCellLow&&...
        | BatUCell<=Table1UCellHigh]
    (junction 44) -> (junction 46) [order 2]
    (junction 45) -> (junction 53) : {LKTFlag=1}
    (junction 46) -> (junction 47) [order 1] : [BatTemp>=Table2TempLow&&...
        | BatTemp<Table2TempHigh&&...
        | BatUCell>=Table2UCellLow&&...
        | BatUCell<=Table2UCellHigh]
    (junction 46) -> (junction 48) [order 2]
    (junction 47) -> (junction 52) : {LKTFlag=2}
    (junction 48) -> (junction 49) [order 1] : [BatTemp>=Table3TempLow&&...
        | BatTemp<Table3TempHigh&&...
        | BatUCell>=Table3UCellLow&&...
        | BatUCell<=Table3UCellHigh]
    (junction 48) -> (junction 50) [order 2] : {LKTFlag=0;}
    (junction 49) -> (junction 51) : {LKTFlag=3;}
    (junction 51) -> (junction 50)
    (junction 52) -> (junction 51)
    (junction 53) -> (junction 52)
    (junction 50) -> (junction 54)
  state ChgCalib
    en:
    SelectedIndex=LocalIndex;
  (default) -> ChgCalibInit
  ChgCalib -> ChgCalibInit
  ChgCalibDelay -> ChgCalibInit [order 1] : [ChargerType<2]
  ChgCalibInit -> ChgCalibDelay : [ChargerType==2]
  ChgCalibDelay -> ChgCalib [order 2] : [TimerOut==1]{LocalIndex=LKTDecide();}
  data: Cycle function_input uint16; Cond function_input uint16; tick local uint8; Timetick local uint8; LKTFlag function_output uint8; SelectedIndex output uint8; BatTemp input; ChargerType input; BatUCell input; Table1TempLow input; Table1TempHigh input; Table1UCellLow input; Table1UCellHigh input; Table2TempLow input; Table2TempHigh input; Table2UCellLow input; Table2UCellHigh input; Table3TempLow input; Table3TempHigh input; Table3UCellLow input; Table3UCellHigh input; TimerOut local boolean; LocalIndex local uint8

== stateflow chart Udan_SOC/SOC_Calculate/UdanSOCCalcn/CapAdder1/Enabled Subsystem1/Chart ==
  state Timer [function]
    state T1 [function]
      state Run(TimeTicks) [function]
        (default) -> (junction 20)
        (junction 20) -> (junction 27) [order 1] : [Init==0]{Init=1;ticks=TimeTicks;}
        (junction 27) -> (junction 29)
        (junction 20) -> (junction 29) [order 2]
        (junction 29) -> (junction 30) [order 2] : {ticks--;}
        (junction 29) -> (junction 31) [order 1] : [ticks<=0]{TimerOut=1;}
      state Clear [function]
        (default) -> (junction 25)
        (junction 25) -> (junction 36) : {Init=0;TimerOut=0;}
    state T2 [function]
      state Run(TimeTicks) [function]
        (default) -> (junction 87)
        (junction 87) -> (junction 88) [order 1] : [Init==0]{Init=1;ticks=TimeTicks;}
        (junction 88) -> (junction 89)
        (junction 87) -> (junction 89) [order 2]
        (junction 89) -> (junction 90) [order 2] : {ticks--;}
        (junction 89) -> (junction 91) [order 1] : [ticks<=0]{Timer2Out=1;}
      state Clear [function]
        (default) -> (junction 99)
        (junction 99) -> (junction 100) : {Init=0;Timer2Out=0;}
  state WaitingSmallCurrent
    en:
    Start_SOC=SOC_STATE_CALCNSOC;
    du:
    Timer.T1.Run(720);
    Timer.T2.Run(240);
    ex:
    Timer.T1.Clear();
    Timer.T2.Clear();
    WaitingSmallCurrent -> WaitingSmallCurrent [order 1] : [Current>80||Current<-80]{Timer.T1.Clear();}
  state WaitingLargeCurrent
    en:
    Start_SOC=SOC_STATE_CALCNSOC;
    du:
    Timer.T1.Run(20);
    ex:
    Timer.T1.Clear();
    WaitingLargeCurrent -> WaitingLargeCurrent [order 1] : [Current>200||Current<-200]{Timer.T1.Clear();}
  state CalibSOC
    en:
    Start_SOC=SOC_STATE_OCVSOC;
    SetLowPower;
  (default) -> WaitingSmallCurrent
  CalibSOC -> WaitingSmallCurrent
  WaitingSmallCurrent -> WaitingLargeCurrent [order 1] : [Timer2Out==1&&...
      | SmallCurrentCalib==0&&0]
  WaitingSmallCurrent -> CalibSOC [order 2] : [TimerOut==1]{SmallCurrentCalib=1;}
  WaitingLargeCurrent -> CalibSOC [order 1] : [TimerOut==1]
  data: TimeTicks function_input uint16; ticks local uint16; Init local boolean; TimeTicks function_input uint16; ticks local uint16; Init local boolean; TimerOut local boolean; Current input; Start_SOC output Enum: SOC_END_CALIB_STATE; SmallCurrentCalib local boolean; Timer2Out local boolean
  events: SetLowPower output FUNCTION_CALL_EVENT

== stateflow chart Udan_SOC/SOC_Calculate/UdanSOCCalcn/CapAdder1/Enabled Subsystem1/Enabled Subsystem1/CalcLeftCap/Chart ==
  state out=abs(in1,in2) [function]
    (default) -> (junction 2)
    (junction 2) -> (junction 7) [order 1] : [in1<in2]
    (junction 7) -> (junction 8) : {out=in2-in1}
    (junction 2) -> (junction 8) [order 2] : {out=in1-in2}
    (junction 8) -> (junction 9)
  (default) -> (junction 28)
  (junction 28) -> (junction 29) [order 1] : [abs(LKTSoc,CalcSoc)<300]
  (junction 28) -> (junction 30) [order 2]
  (junction 29) -> (junction 37) : {SocOut=CalcSoc;}
  (junction 30) -> (junction 31) [order 1] : [abs(LKTSoc,CalcSoc)>=300&&...
      | LKTSoc>CalcSoc&&LKTSoc>300]
  (junction 30) -> (junction 32) [order 2]
  (junction 31) -> (junction 36) : {SocOut=LKTSoc-300;}
  (junction 32) -> (junction 33) [order 1] : [abs(LKTSoc,CalcSoc)>=300&&...
      | LKTSoc<CalcSoc]
  (junction 32) -> (junction 34) [order 2] : {SocOut=CalcSoc;}
  (junction 33) -> (junction 35) : {SocOut=LKTSoc+300;}
  (junction 35) -> (junction 34)
  (junction 36) -> (junction 35)
  (junction 37) -> (junction 36)
  (junction 34) -> (junction 38)
  data: in1 function_input uint16; in2 function_input uint16; out function_output uint16; LKTSoc input; CalcSoc input; SocOut output uint16
